simulink model "PaceMaker_Simulink_Model"  (R2018b)
settings: Solver=FixedStepAuto  StartTime=0.0  StopTime=inf  FixedStep=1e-3  RelTol=1e-3  EnableMultiTasking=on
undefined symbols (not defined in the file): A0, A1, D0, D1, D10, D11, D12, D13, D2, D3, D5, D6, D8, D9, PTA0, PTA1, PTA2, PTB2, PTB3, PTB9, PTC16, PTC17, PTC2, PTC4, PTD0, PTD1, PTD2, PTD3
libraries: frdmk64flib x21
(part 1 of 2)
settings Model: ExtModeTrigDuration=5  Creator=elgendya  LastModifiedBy=abdul
settings SolverCC: AutoInsertRateTranBlk=on
settings DataIOCC: LimitDataPoints=on
settings OptimizationCC: PassReuseOutputArgsAs=Individual arguments  MaxStackSize=64
settings DebuggingCC: ParameterTunabilityLossMsg=error  AllowSymbolicDim=off  SFUnexpectedBacktrackingDiag=warning  SFNoUnconditionalDefaultTransitionDiag=warning  SFExecutionAtInitializationDiag=none
settings HardwareCC: ProdBitPerPointer=32  ProdBitPerSizeT=32  ProdBitPerPtrDiffT=32  ProdLargestAtomicInteger=Long  ProdLargestAtomicFloat=Double  ProdWordSize=32  ProdHWDeviceType=ARM Compatible->ARM Cortex
settings SFSimCC: SimUseLocalCustomCode=off  MATLABDynamicMemAlloc=off
settings RTWCC: SystemTargetFile=ert.tlc  HardwareBoard=NXP FRDM-K64F  TLCOptions="-aInlineSetEventsForThisBaseRateFcn=TLC_FALSE -aSuppressMultiTaskScheduler=TLC_FALSE    -aRateBasedStepFcn=0"  TemplateMakefile=ert_default_tmf  GenerateReport=on  RTWUseLocalCustomCode=off  Toolchain=GNU Tools for ARM Embedded Processors  IncludeHyperlinkInReport=on  LaunchReport=on  GenerateTraceInfo=on  GenerateTraceReport=on  GenerateTraceReportSl=on  GenerateTraceReportSf=on  GenerateTraceReportEml=on
settings CodeAppCC: ForceParamTrailComments=on  IgnoreCustomStorageClasses=off  OperatorAnnotations=on  SimulinkDataObjDesc=on  SFDataObjDesc=on  InsertBlockDesc=on
settings ConfigComp: CovMetricSettings=dw  CovHtmlReporting=on  CovSaveCumulativeToWorkspaceVar=on  CovSaveSingleToWorkspaceVar=on  CovShowResultsExplorer=off  CovExternalEMLEnable=off  CovSFcnEnable=off

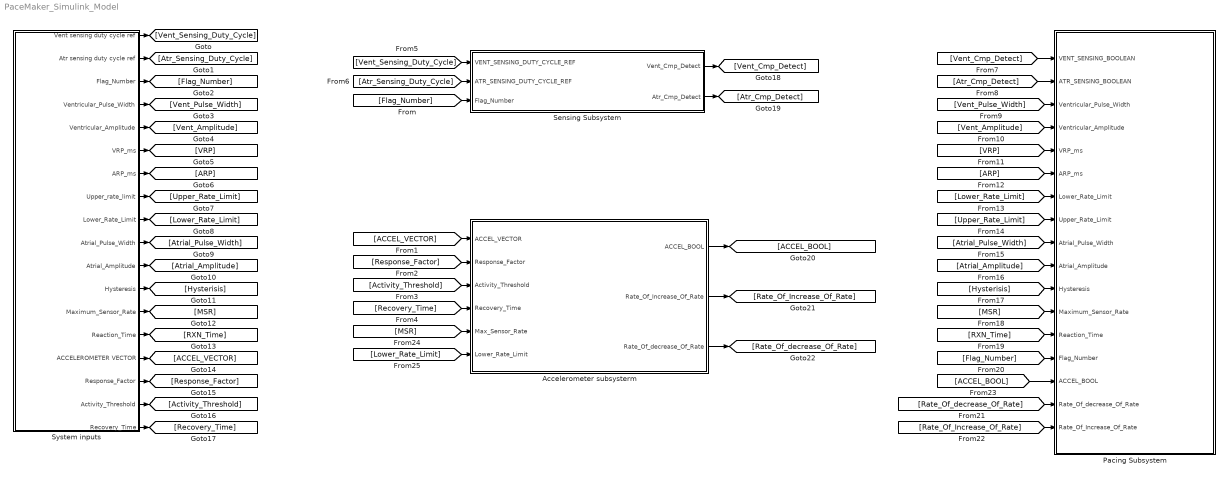
== system PaceMaker_Simulink_Model ==
  "Accelerometer subsysterm " : Subsystem
  "Pacing Subsystem " : Subsystem
  Sensing Subsystem : Subsystem
  "System inputs " : Subsystem
  wires:
  "System inputs "/1(Vent sensing duty cycle ref) -> [Vent_Sensing_Duty_Cycle]
  "System inputs "/2("Atr sensing duty cycle ref ") -> [Atr_Sensing_Duty_Cycle]
  "System inputs "/3(Flag_Number) -> [Flag_Number]
  "System inputs "/4(Ventricular_Pulse_Width) -> [Vent_Pulse_Width]
  "System inputs "/5(Ventricular_Amplitude) -> [Vent_Amplitude]
  "System inputs "/6(VRP_ms) -> [VRP]
  "System inputs "/7(ARP_ms) -> [ARP]
  "System inputs "/8(Upper_rate_limit) -> [Upper_Rate_Limit]
  "System inputs "/9(Lower_Rate_Limit) -> [Lower_Rate_Limit]
  "System inputs "/10(Atrial_Pulse_Width) -> [Atrial_Pulse_Width]
  "System inputs "/11(Atrial_Amplitude) -> [Atrial_Amplitude]
  "System inputs "/12(Hysteresis) -> [Hysterisis]
  "System inputs "/13(Maximum_Sensor_Rate) -> [MSR]
  "System inputs "/14(Reaction_Time) -> [RXN_Time]
  "System inputs "/15(ACCELEROMETER VECTOR) -> [ACCEL_VECTOR]
  "System inputs "/16(Response_Factor) -> [Response_Factor]
  "System inputs "/17(Activity_Threshold) -> [Activity_Threshold]
  "System inputs "/18(Recovery_Time) -> [Recovery_Time]
  [Flag_Number] -> Sensing Subsystem/3(" Flag_Number")
  [ACCEL_VECTOR] -> "Accelerometer subsysterm "/1(ACCEL_VECTOR)
  [Response_Factor] -> "Accelerometer subsysterm "/2(Response_Factor)
  [Activity_Threshold] -> "Accelerometer subsysterm "/3("Activity_Threshold ")
  [Recovery_Time] -> "Accelerometer subsysterm "/4(Recovery_Time)
  [Vent_Sensing_Duty_Cycle] -> Sensing Subsystem/1(" VENT_SENSING_DUTY_CYCLE_REF")
  [Atr_Sensing_Duty_Cycle] -> Sensing Subsystem/2(" ATR_SENSING_DUTY_CYCLE_REF")
  Sensing Subsystem/1(Vent_Cmp_Detect) -> [Vent_Cmp_Detect]
  Sensing Subsystem/2(Atr_Cmp_Detect) -> [Atr_Cmp_Detect]
  [Vent_Cmp_Detect] -> "Pacing Subsystem "/1(VENT_SENSING_BOOLEAN)
  [Atr_Cmp_Detect] -> "Pacing Subsystem "/2(ATR_SENSING_BOOLEAN)
  [Vent_Pulse_Width] -> "Pacing Subsystem "/3(Ventricular_Pulse_Width)
  [Vent_Amplitude] -> "Pacing Subsystem "/4(Ventricular_Amplitude)
  [VRP] -> "Pacing Subsystem "/5(VRP_ms)
  [ARP] -> "Pacing Subsystem "/6(ARP_ms)
  [Lower_Rate_Limit] -> "Pacing Subsystem "/7(Lower_Rate_Limit)
  [Upper_Rate_Limit] -> "Pacing Subsystem "/8(Upper_Rate_Limit)
  [Atrial_Pulse_Width] -> "Pacing Subsystem "/9(Atrial_Pulse_Width)
  [Atrial_Amplitude] -> "Pacing Subsystem "/10(Atrial_Amplitude)
  [Hysterisis] -> "Pacing Subsystem "/11(Hysteresis)
  [MSR] -> "Pacing Subsystem "/12(Maximum_Sensor_Rate)
  [RXN_Time] -> "Pacing Subsystem "/13(Reaction_Time)
  [Flag_Number] -> "Pacing Subsystem "/14(Flag_Number)
  "Accelerometer subsysterm "/1(ACCEL_BOOL) -> [ACCEL_BOOL]
  "Accelerometer subsysterm "/2(Rate_Of_Increase_Of_Rate) -> [Rate_Of_Increase_Of_Rate]
  "Accelerometer subsysterm "/3(Rate_Of_decrease_Of_Rate) -> [Rate_Of_decrease_Of_Rate]
  [Rate_Of_decrease_Of_Rate] -> "Pacing Subsystem "/16(Rate_Of_decrease_Of_Rate)
  [Rate_Of_Increase_Of_Rate] -> "Pacing Subsystem "/17(Rate_Of_Increase_Of_Rate)
  [ACCEL_BOOL] -> "Pacing Subsystem "/15(ACCEL_BOOL)
  [MSR] -> "Accelerometer subsysterm "/5(Max_Sensor_Rate)
  [Lower_Rate_Limit] -> "Accelerometer subsysterm "/6(Lower_Rate_Limit)

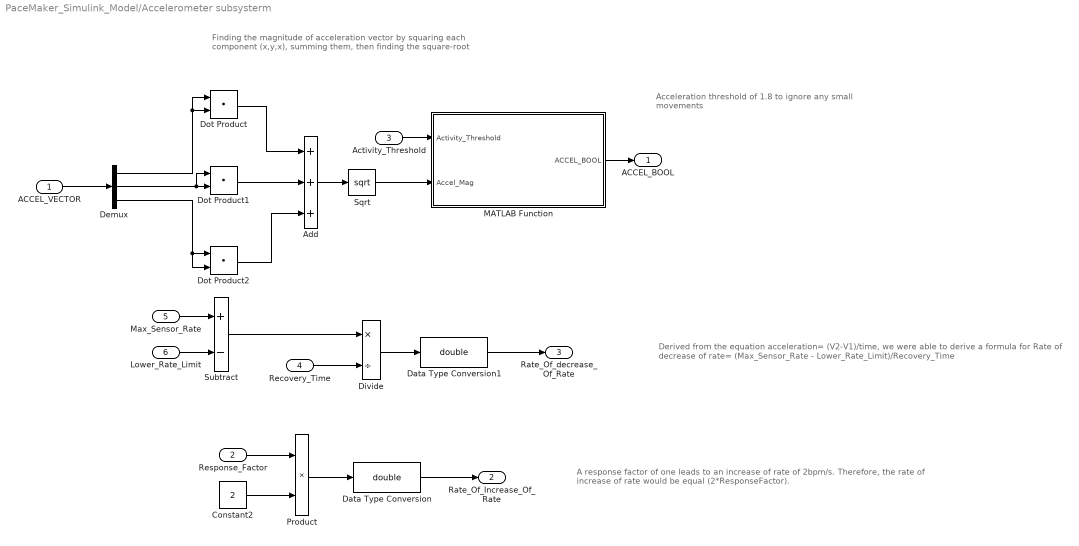
== system PaceMaker_Simulink_Model/Accelerometer subsysterm  ==
  note: Finding the magnitude of acceleration vector by squaring each
      | component (x,y,x), summing them, then finding the square-root
  note: Acceleration threshold of 1.8 to ignore any
      | small movements
  note: A response factor of one leads to an increase of rate of 2bpm/s. Therefore,
      | the rate of increase of rate would be equal (2*ResponseFactor).
  note: Derived from the equation acceleration= (V2-V1)/time, we were able to derive
      | a formula for Rate of decrease of rate= (Max_Sensor_Rate - Lower_Rate_Limit)/Recovery_Time
  ACCEL_VECTOR : Inport
  Response_Factor : Inport  Port=2  OutDataTypeStr=uint16
  "Activity_Threshold " : Inport  Port=3
  Recovery_Time : Inport  Port=4  OutDataTypeStr=uint16
  Max_Sensor_Rate : Inport  Port=5
  Lower_Rate_Limit : Inport  Port=6
  Add : Sum  Inputs=+++
  Constant2 : Constant  Value=2  OutDataTypeStr=uint16
  Data Type Conversion : DataTypeConversion  OutDataTypeStr=double
  Data Type Conversion1 : DataTypeConversion  OutDataTypeStr=double
  Demux : Demux  Outputs=3
  Divide : Product  Inputs=*/
  Dot Product : DotProduct  InputSameDT=on  OutDataTypeStr=Inherit: Inherit via internal rule
  Dot Product1 : DotProduct  InputSameDT=on  OutDataTypeStr=Inherit: Inherit via internal rule
  Dot Product2 : DotProduct  InputSameDT=on  OutDataTypeStr=Inherit: Inherit via internal rule
  MATLAB Function : MATLAB Function  TreatAsAtomicUnit=on
  Product : Product  OutDataTypeStr=uint16
  Sqrt : Sqrt  SaturateOnIntegerOverflow=on
  Subtract : Sum  Inputs=+-
  ACCEL_BOOL : Outport
  Rate_Of_Increase_Of_Rate : Outport  Port=2  OutDataTypeStr=double
  Rate_Of_decrease_Of_Rate : Outport  Port=3  OutDataTypeStr=double
  wires:
  ACCEL_VECTOR/1 -> Demux/1
  Demux/3 -> Dot Product2/1, Dot Product2/2
  Demux/2 -> Dot Product1/1, Dot Product1/2
  Demux/1 -> Dot Product/2, Dot Product/1
  Dot Product1/1 -> Add/2
  Dot Product/1 -> Add/1
  Dot Product2/1 -> Add/3
  Add/1 -> Sqrt/1
  Response_Factor/1 -> Product/1
  Constant2/1 -> Product/2
  "Activity_Threshold "/1 -> MATLAB Function/1(Activity_Threshold)
  Recovery_Time/1 -> Divide/2
  Product/1 -> Data Type Conversion/1
  Data Type Conversion/1 -> Rate_Of_Increase_Of_Rate/1
  Divide/1 -> Data Type Conversion1/1
  Data Type Conversion1/1 -> Rate_Of_decrease_Of_Rate/1
  Lower_Rate_Limit/1 -> Subtract/2
  Max_Sensor_Rate/1 -> Subtract/1
  Subtract/1 -> Divide/1
  Sqrt/1 -> MATLAB Function/2(Accel_Mag)
  MATLAB Function/1(ACCEL_BOOL) -> ACCEL_BOOL/1

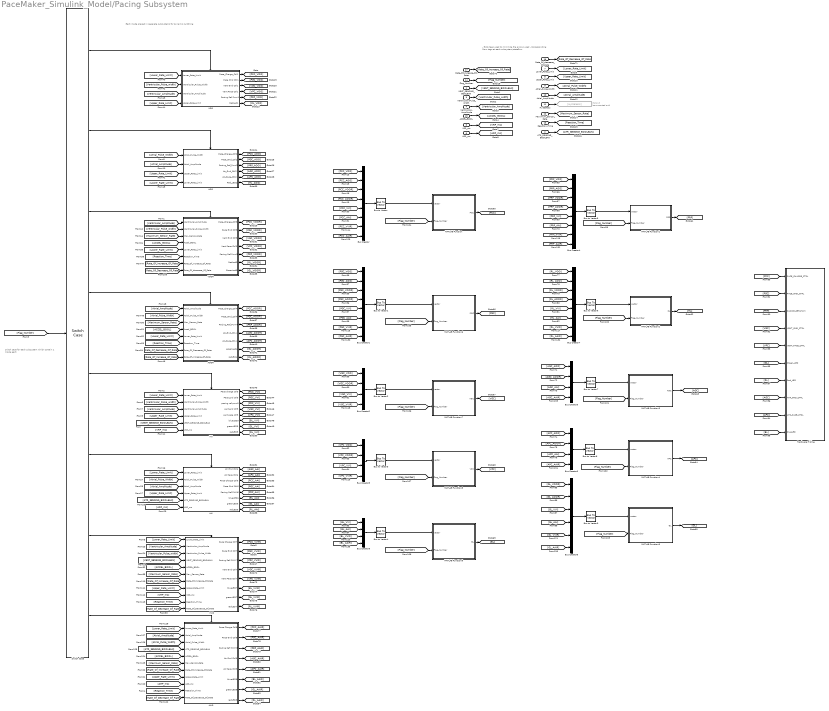
== system PaceMaker_Simulink_Model/Pacing Subsystem  ==
  note: - Goto tags used to minimize the arrows used
      | - Corresponding From tags at each subsystem/stateflow
  note: switch case for each subsystem which contain
      | 1 mode each
  note: Each mode placed in separate subsystems for dynamic switching
  VENT_SENSING_BOOLEAN : Inport
  ATR_SENSING_BOOLEAN : Inport  Port=2
  Ventricular_Pulse_Width : Inport  Port=3
  Ventricular_Amplitude : Inport  Port=4  OutDataTypeStr=uint16
  VRP_ms : Inport  Port=5
  ARP_ms : Inport  Port=6
  Lower_Rate_Limit : Inport  Port=7
  Upper_Rate_Limit : Inport  Port=8
  Atrial_Pulse_Width : Inport  Port=9
  Atrial_Amplitude : Inport  Port=10  OutDataTypeStr=uint16
  Hysteresis : Inport  Port=11
  Maximum_Sensor_Rate : Inport  Port=12
  Reaction_Time : Inport  Port=13
  Flag_Number : Inport  Port=14
  ACCEL_BOOL : Inport  Port=15
  Rate_Of_decrease_Of_Rate : Inport  Port=16
  Rate_Of_Increase_Of_Rate : Inport  Port=17
  AAI : Subsystem  TreatAsAtomicUnit=on
  AAIR : Subsystem  TreatAsAtomicUnit=on
  AOO : Subsystem  TreatAsAtomicUnit=on
  AOOR : Subsystem  TreatAsAtomicUnit=on
  Bus Creator{,1,4,7} (4 alike) : BusCreator  Inputs=8
  Bus Creator{2..3,5..6,9} (5 alike) : BusCreator  Inputs=4
  Bus Creator8 : BusCreator  Inputs=6
  Bus to Vector{,1..9} (10 alike) : BusToVector
  Goto13 : Goto  Commented=on  GotoTag=Hysteresis
  Hardware Hiding : Subsystem  TreatAsAtomicUnit=on
  MATLAB Function : MATLAB Function  TreatAsAtomicUnit=on
  MATLAB Function1 : MATLAB Function  TreatAsAtomicUnit=on
  MATLAB Function2 : MATLAB Function  TreatAsAtomicUnit=on
  MATLAB Function3 : MATLAB Function  TreatAsAtomicUnit=on
  MATLAB Function4 : MATLAB Function  TreatAsAtomicUnit=on
  MATLAB Function5 : MATLAB Function  TreatAsAtomicUnit=on
  MATLAB Function6 : MATLAB Function  TreatAsAtomicUnit=on
  MATLAB Function7 : MATLAB Function  TreatAsAtomicUnit=on
  MATLAB Function8 : MATLAB Function  TreatAsAtomicUnit=on
  MATLAB Function9 : MATLAB Function  TreatAsAtomicUnit=on
  Switch Case : SwitchCase  CaseConditions={1,2,3,4,5,6,7,8,}  ShowDefaultCase=off
  VOO : Subsystem  TreatAsAtomicUnit=on
  VOOR : Subsystem  TreatAsAtomicUnit=on
  "VVI " : Subsystem  TreatAsAtomicUnit=on
  VVIR : Subsystem  TreatAsAtomicUnit=on
  wires:
  VRP_ms/1 -> [VRP_ms]
  ACCEL_BOOL/1 -> [ACCEL_BOOL]
  Ventricular_Amplitude/1 -> [Ventricular_Amplitude]
  Ventricular_Pulse_Width/1 -> [Ventricular_Pulse_width]
  VENT_SENSING_BOOLEAN/1 -> [VENT_SENSING_BOOLEAN]
  ARP_ms/1 -> [ARP_ms]
  Lower_Rate_Limit/1 -> [Lower_Rate_Limit]
  Upper_Rate_Limit/1 -> [Upper_Rate_Limit]
  Atrial_Pulse_Width/1 -> [Atrial_Pulse_Width]
  Atrial_Amplitude/1 -> [Atrial_Amplitude]
  Hysteresis/1 -> Goto13/1
  Maximum_Sensor_Rate/1 -> [Maximum_Sensor_Rate]
  Reaction_Time/1 -> [Reaction_Time]
  Switch Case/1 -> VOO/Action
  Switch Case/2 -> AOO/Action
  Switch Case/4 -> AOOR/Action
  Switch Case/5 -> "VVI "/Action
  Switch Case/6 -> AAI/Action
  Switch Case/7 -> VVIR/Action
  [Lower_Rate_Limit] -> VOO/1(Lower_Rate_LImit)
  [Ventricular_Pulse_width] -> VOO/2(Ventricular_Pulse_Width)
  [Ventricular_Amplitude] -> VOO/3(Ventricular_Amplitude)
  [Upper_Rate_Limit] -> VOO/4(Upper_Rate_Limit)
  [Atrial_Pulse_Width] -> AOO/1(Atrial_Pulse_Width)
  [Atrial_Amplitude] -> AOO/2(Atrial_Amplitude)
  [Lower_Rate_Limit] -> AOO/4(Lower_Rate_Limit)
  [Upper_Rate_Limit] -> AOO/3(Upper_Rate_Limit)
  [Ventricular_Amplitude] -> VOOR/1(Ventricular_Amplitude)
  [Maximum_Sensor_Rate] -> VOOR/3(Max_Sensor_Rate)
  [Ventricular_Pulse_width] -> VOOR/2(Ventricular_Pulse_Width)
  [ACCEL_BOOL] -> VOOR/4(Accel_BOOL)
  [Lower_Rate_Limit] -> VOOR/5(Lower_Rate_Limit)
  [Reaction_Time] -> VOOR/6(Reaction_Time)
  [Atrial_Amplitude] -> AOOR/1(Atrial_Amplitude)
  [Maximum_Sensor_Rate] -> AOOR/3(Max_Sensor_Rate)
  [Atrial_Pulse_Width] -> AOOR/2(Atrial_Pulse_Width)
  [ACCEL_BOOL] -> AOOR/4(Accel_BOOL)
  [Lower_Rate_Limit] -> AOOR/5(Lower_Rate_Limit)
  [Reaction_Time] -> AOOR/6(Reaction_Time)
  [Lower_Rate_Limit] -> "VVI "/1(Lower_Rate_LImit)
  [Ventricular_Pulse_width] -> "VVI "/2(Ventricular_Pulse_Width)
  [Ventricular_Amplitude] -> "VVI "/3(Ventricular_Amplitude)
  [Upper_Rate_Limit] -> "VVI "/4(Upper_Rate_Limit)
  [VENT_SENSING_BOOLEAN] -> "VVI "/5(VENT_SENSING_BOOLEAN)
  [VRP_ms] -> "VVI "/6(VRP_ms)
  ATR_SENSING_BOOLEAN/1 -> [ATR_SENSING_BOOLEAN]
  [Lower_Rate_Limit] -> AAI/1(Lower_Rate_Limit)
  [Upper_Rate_Limit] -> AAI/4(Upper_Rate_Limit)
  [ATR_SENSING_BOOLEAN] -> AAI/5(ATR_SENSING_BOOLEAN)
  [Atrial_Pulse_Width] -> AAI/2(Atrial_Pulse_Width)
  [Atrial_Amplitude] -> AAI/3(Atrial_Amplitude)
  [ARP_ms] -> AAI/6(ARP_ms)
  Flag_Number/1 -> [Flag_Number]
  [Flag_Number] -> Switch Case/1
  VOO/1(Pace_Charge_Ctrl1) -> [PCC_VOO]
  VOO/2(Pace Gnd Ctrl1) -> [PGC_VOO]
  VOO/3(Vent Gnd Ctrl1) -> [VGC_VOO]
  VOO/4(Vent Pace Ctrl1) -> [VPC_VOO]
  VOO/5(Pacing Ref Pwm1) -> [PRP_VOO]
  VOO/6(RedLed1) -> [RL_VOO]
  AOO/1(Pace_Charge_Ctrl2) -> [PCC_AOO]
  AOO/2(Pace_Gnd_Ctrl2) -> [PGC_AOO]
  AOO/3(Pacing_Ref_Pwm2) -> [PRP_AOO]
  AOO/4(Atr_Gnd_Ctrl2) -> [AGC_AOO]
  AOO/5(Atr_Pace_Ctrl2) -> [APC_AOO]
  VOOR/1(Pace_Charge_Ctrl3) -> [PCC_VOOR]
  VOOR/2(Pace Gnd Ctrl3) -> [PGC_VOOR]
  VOOR/3(Vent Gnd Ctrl3) -> [VGC_VOOR]
  VOOR/4(Vent Pace Ctrl3) -> [VPC_VOOR]
  VOOR/5(Pacing Ref Pwm3) -> [PRP_VOOR]
  VOOR/7(GreenLed3) -> [GL_VOOR]
  VOOR/6(RedLed3) -> [RL_VOOR]
  AOOR/1(Pace_Charge_Ctrl4) -> [PCC_AOOR]
  AOOR/2(Pace_Gnd_Ctrl4) -> [PGC_AOOR]
  AOOR/3(Pacing_Ref_Pwm4) -> [PRP_AOOR]
  AOOR/4(Atr_Gnd_Ctrl4) -> [AGC_AOOR]
  AOOR/5(Atr_Pace_Ctrl4) -> [APC_AOOR]
  AOOR/6(greenLed4) -> [GL_AOOR]
  AOOR/7(redLEd4) -> [RL_AOOR]
  "VVI "/1(Pace charge ctrl5) -> [PCC_VVI]
  "VVI "/2(Pace gnd ctrl5) -> [PGC_VVI]
  "VVI "/3(pacing ref pwm5) -> [PRP_VVI]
  "VVI "/4(vent gnd ctrl5) -> [VGC_VVI]
  "VVI "/5(vent pace ctrl5) -> [VPC_VVI]
  "VVI "/6(blueLED5) -> [BL_VVI]
  "VVI "/7(greenLED5) -> [GL_VVI]
  "VVI "/8(redLED5) -> [RL_VVI]
  AAI/1(Atr Gnd Ctrl6) -> [AGC_AAI]
  AAI/2(Atr Pace Ctrl6) -> [APC_AAI]
  AAI/3(Pace Charge Ctrl6) -> [PCC_AAI]
  AAI/5(Pacing Ref PWM6) -> [PRP_AAI]
  AAI/6(blueLED6) -> [BL_AAI]
  AAI/7(greenLED6) -> [GL_AAI]
  AAI/8(redLED6) -> [RL_AAI]
  AAI/4(Pace Gnd Ctrl6) -> [PGC_AAI]
  [PCC_VOO] -> Bus Creator/1
  [PCC_AOO] -> Bus Creator/2
  [PCC_VOOR] -> Bus Creator/3
  [PCC_AOOR] -> Bus Creator/4
  [PCC_VVI] -> Bus Creator/5
  [PCC_AAI] -> Bus Creator/6
  [PGC_AAI] -> Bus Creator1/6
  [PGC_VVI] -> Bus Creator1/5
  [PGC_AOOR] -> Bus Creator1/4
  [PGC_VOOR] -> Bus Creator1/3
  [PGC_AOO] -> Bus Creator1/2
  [PGC_VOO] -> Bus Creator1/1
  [VGC_VOO] -> Bus Creator2/1
  [VGC_VOOR] -> Bus Creator2/2
  [VGC_VVI] -> Bus Creator2/3
  [VPC_VVI] -> Bus Creator3/3
  [VPC_VOOR] -> Bus Creator3/2
  [VPC_VOO] -> Bus Creator3/1
  [PRP_AAI] -> Bus Creator4/6
  [PRP_VVI] -> Bus Creator4/5
  [PRP_AOOR] -> Bus Creator4/4
  [PRP_VOOR] -> Bus Creator4/3
  [PRP_AOO] -> Bus Creator4/2
  [PRP_VOO] -> Bus Creator4/1
  [AGC_AAI] -> Bus Creator5/3
  [AGC_AOOR] -> Bus Creator5/2
  [AGC_AOO] -> Bus Creator5/1
  [APC_AOO] -> Bus Creator6/1
  [APC_AOOR] -> Bus Creator6/2
  [APC_AAI] -> Bus Creator6/3
  AOO/6(Red_LED2) -> [RL_AOO]
  [RL_VOO] -> Bus Creator7/1
  [RL_AOO] -> Bus Creator7/2
  [RL_VOOR] -> Bus Creator7/3
  [RL_AOOR] -> Bus Creator7/4
  [RL_VVI] -> Bus Creator7/5
  [RL_AAI] -> Bus Creator7/6
  [GL_VOOR] -> Bus Creator8/1
  [GL_AOOR] -> Bus Creator8/2
  [GL_VVI] -> Bus Creator8/3
  [GL_AAI] -> Bus Creator8/4
  [BL_VVI] -> Bus Creator9/1
  [BL_AAI] -> Bus Creator9/2
  Bus Creator/1 -> Bus to Vector/1
  Bus Creator1/1 -> Bus to Vector1/1
  Bus Creator2/1 -> Bus to Vector2/1
  Bus Creator3/1 -> Bus to Vector3/1
  Bus Creator9/1 -> Bus to Vector4/1
  Bus Creator4/1 -> Bus to Vector5/1
  Bus Creator7/1 -> Bus to Vector6/1
  Bus Creator5/1 -> Bus to Vector7/1
  Bus Creator6/1 -> Bus to Vector8/1
  Bus Creator8/1 -> Bus to Vector9/1
  Bus to Vector/1 -> MATLAB Function/1(vector)
  MATLAB Function/1(PCC) -> [PCC]
  MATLAB Function1/1(PRP) -> [PRP]
  Bus to Vector5/1 -> MATLAB Function1/1(vector)
  Bus to Vector6/1 -> MATLAB Function2/1(vector)
  MATLAB Function2/1(RL) -> [RL]
  MATLAB Function3/1(AGC) -> [AGC]
  Bus to Vector7/1 -> MATLAB Function3/1(vector)
  Bus to Vector8/1 -> MATLAB Function4/1(vector)
  MATLAB Function4/1(APC) -> [APC]
  MATLAB Function5/1(GL) -> [GL]
  Bus to Vector9/1 -> MATLAB Function5/1(vector)
  [PCC] -> Hardware Hiding/1(PACE_CHARGE_CTRL)
  [PRP] -> Hardware Hiding/3(PACING_REF_PWM)
  [PGC] -> Hardware Hiding/2(PACE_GND_CTRL)
  [VGC] -> Hardware Hiding/4(VENT_GND_CTRL)
  [VPC] -> Hardware Hiding/5(VENT_PACE_CTRL)
  [APC] -> Hardware Hiding/9(ATR_PACE_CTRL)
  [GL] -> Hardware Hiding/6(Green_LED)
  [AGC] -> Hardware Hiding/8(ATR_GND_CTRL)
  [RL] -> Hardware Hiding/7(Red_LED)
  [BL] -> Hardware Hiding/10(blueLED)
  [Flag_Number] -> MATLAB Function1/2(Flag_Number)
  [Flag_Number] -> MATLAB Function2/2(Flag_Number)
  [Flag_Number] -> MATLAB Function3/2(Flag_Number)
  [Flag_Number] -> MATLAB Function4/2(Flag_Number)
  [Flag_Number] -> MATLAB Function5/2(Flag_Number)
  [Flag_Number] -> MATLAB Function/2(Flag_Number)
  [Flag_Number] -> MATLAB Function6/2(Flag_Number)
  MATLAB Function6/1(PGC) -> [PGC]
  Bus to Vector1/1 -> MATLAB Function6/1(vector)
  MATLAB Function7/1(VGC) -> [VGC]
  [Flag_Number] -> MATLAB Function7/2(Flag_Number)
  [Flag_Number] -> MATLAB Function8/2(Flag_Number)
  MATLAB Function8/1(VPC) -> [VPC]
  Bus to Vector3/1 -> MATLAB Function8/1(vector)
  Bus to Vector4/1 -> MATLAB Function9/1(vector)
  MATLAB Function9/1(BL) -> [BL]
  [Flag_Number] -> MATLAB Function9/2(Flag_Number)
  Bus to Vector2/1 -> MATLAB Function7/1(vector)
  [Rate_Of_Increase_Of_Rate] -> VOOR/7(Rate_Of_Increase_Of_Rate)
  [Rate_Of_Decrease_Of_Rate] -> VOOR/8(Rate_Of_decrease_Of_Rate)
  Rate_Of_decrease_Of_Rate/1 -> [Rate_Of_Decrease_Of_Rate]
  Rate_Of_Increase_Of_Rate/1 -> [Rate_Of_Increase_Of_Rate]
  [Rate_Of_Increase_Of_Rate] -> AOOR/8(Rate_Of_increase_Of_Rate)
  [Rate_Of_Decrease_Of_Rate] -> AOOR/7(Rate_Of_Decrease_Of_Rate)
  [Lower_Rate_Limit] -> VVIR/1(Lower_Rate_Limit)
  [Ventricular_Amplitude] -> VVIR/2(Ventricular_Amplitude)
  [Ventricular_Pulse_width] -> VVIR/3(Ventricular_Pulse_Width)
  [VENT_SENSING_BOOLEAN] -> VVIR/4(VENT_SENSING_BOOLEAN)
  [ACCEL_BOOL] -> VVIR/5(ACCEL_BOOL)
  [Maximum_Sensor_Rate] -> VVIR/6(Max_Sensor_Rate)
  [Rate_Of_Increase_Of_Rate] -> VVIR/7(Rate_Of_Increase_Of_Rate)
  [Upper_Rate_Limit] -> VVIR/8(Upper_Rate_Limit)
  [VRP_ms] -> VVIR/9(VRP_ms)
  [Reaction_Time] -> VVIR/10(Reaction_Time)
  VVIR/1(Pace Charge Ctrl7) -> [PCC_VVIR]
  VVIR/2(Pace Gnd Ctrl7) -> [PGC_VVIR]
  VVIR/3(Pacing Ref PWM 7) -> [PRP_VVIR]
  VVIR/4(Vent Gnd Ctrl7) -> [VGC_VVIR]
  VVIR/5(Vent Pace Ctrl7) -> [VPC_VVIR]
  VVIR/6(blueLED7) -> [BL_VVIR]
  VVIR/7(greenLED7) -> [GL_VVIR]
  VVIR/8(redLED7) -> [RL_VVIR]
  [PCC_VVIR] -> Bus Creator/7
  [PGC_VVIR] -> Bus Creator1/7
  [PRP_VVIR] -> Bus Creator4/7
  [RL_VVIR] -> Bus Creator7/7
  [VGC_VVIR] -> Bus Creator2/4
  [VPC_VVIR] -> Bus Creator3/4
  [BL_VVIR] -> Bus Creator9/3
  [GL_VVIR] -> Bus Creator8/5
  Switch Case/3 -> VOOR/Action
  Switch Case/8 -> AAIR/Action
  [Reaction_Time] -> AAIR/10(Reaction_Time)
  [ARP_ms] -> AAIR/9(ARP_ms)
  [Upper_Rate_Limit] -> AAIR/8(Upper_Rate_Limit)
  [Rate_Of_Increase_Of_Rate] -> AAIR/7(Rate_Of_Increase_Of_Rate)
  [Rate_Of_Decrease_Of_Rate] -> VVIR/11(Rate_Of_Decrease_Of_Rate)
  [Rate_Of_Decrease_Of_Rate] -> AAIR/11(Rate_Of_Decrease_Of_Rate)
  [Maximum_Sensor_Rate] -> AAIR/6(Max_Sensor_Rate)
  [ACCEL_BOOL] -> AAIR/5(ACCEL_BOOL)
  [ATR_SENSING_BOOLEAN] -> AAIR/4(ATR_SENSING_BOOLEAN)
  [Atrial_Pulse_Width] -> AAIR/3(Atrial_Pulse_Width)
  [Atrial_Amplitude] -> AAIR/2(Atrial_Amplitude)
  [Lower_Rate_Limit] -> AAIR/1(Lower_Rate_Limit)
  AAIR/1(Pace Charge Ctrl8) -> [PCC_AAIR]
  AAIR/2(Pace Gnd Ctrl8) -> [PGC_AAIR]
  AAIR/3(Pacing Ref PWM 8) -> [PRP_AAIR]
  AAIR/4(Atr Gnd Ctrl8) -> [AGC_AAIR]
  AAIR/5(Atr Pace Ctrl8) -> [APC_AAIR]
  AAIR/6(blueLED8) -> [BL_AAIR]
  AAIR/7(greenLED8) -> [GL_AAIR]
  AAIR/8(redLED8) -> [RL_AAIR]
  [PCC_AAIR] -> Bus Creator/8
  [PGC_AAIR] -> Bus Creator1/8
  [PRP_AAIR] -> Bus Creator4/8
  [RL_AAIR] -> Bus Creator7/8
  [AGC_AAIR] -> Bus Creator5/4
  [APC_AAIR] -> Bus Creator6/4
  [BL_AAIR] -> Bus Creator9/4
  [GL_AAIR] -> Bus Creator8/6

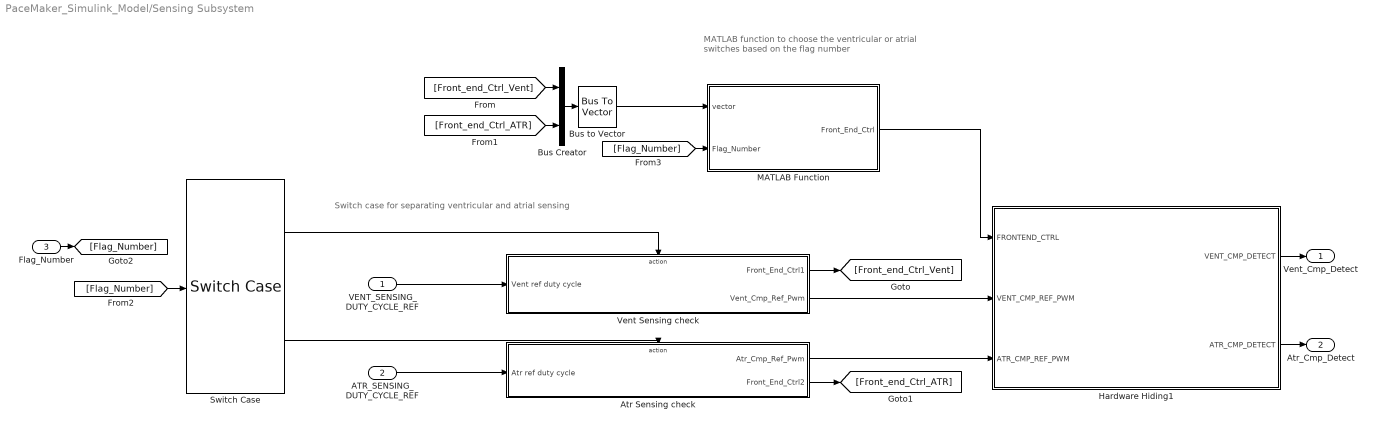
== system PaceMaker_Simulink_Model/Sensing Subsystem ==
  note: Switch case for separating ventricular and atrial sensing
  note: MATLAB function to choose the ventricular or
      | atrial switches based on the flag number
  " VENT_SENSING_DUTY_CYCLE_REF" : Inport
  " ATR_SENSING_DUTY_CYCLE_REF" : Inport  Port=2
  " Flag_Number" : Inport  Port=3
  Atr Sensing check : Subsystem  TreatAsAtomicUnit=on
  Bus Creator : BusCreator  Inputs=2
  Bus to Vector : BusToVector
  Hardware Hiding1 : Subsystem
  MATLAB Function : MATLAB Function  TreatAsAtomicUnit=on
  Switch Case : SwitchCase  CaseConditions={[5,7],[6,8]}  ShowDefaultCase=off
  Vent Sensing check : Subsystem  TreatAsAtomicUnit=on
  Vent_Cmp_Detect : Outport
  Atr_Cmp_Detect : Outport  Port=2
  wires:
  Switch Case/1 -> Vent Sensing check/Action
  " VENT_SENSING_DUTY_CYCLE_REF"/1 -> Vent Sensing check/1("Vent ref duty cycle ")
  Switch Case/2 -> Atr Sensing check/Action
  " ATR_SENSING_DUTY_CYCLE_REF"/1 -> Atr Sensing check/1("Atr ref duty cycle ")
  Vent Sensing check/2(Vent_Cmp_Ref_Pwm) -> Hardware Hiding1/2(VENT_CMP_REF_PWM)
  Hardware Hiding1/1(VENT_CMP_DETECT) -> Vent_Cmp_Detect/1
  Atr Sensing check/1(Atr_Cmp_Ref_Pwm) -> Hardware Hiding1/3(ATR_CMP_REF_PWM)
  Hardware Hiding1/2(ATR_CMP_DETECT) -> Atr_Cmp_Detect/1
  Vent Sensing check/1(Front_End_Ctrl1) -> [Front_end_Ctrl_Vent]
  Atr Sensing check/2(Front_End_Ctrl2) -> [Front_end_Ctrl_ATR]
  [Front_end_Ctrl_Vent] -> Bus Creator/1
  [Front_end_Ctrl_ATR] -> Bus Creator/2
  Bus Creator/1 -> Bus to Vector/1
  Bus to Vector/1 -> MATLAB Function/1(vector)
  " Flag_Number"/1 -> [Flag_Number]
  [Flag_Number] -> Switch Case/1
  [Flag_Number] -> MATLAB Function/2(Flag_Number)
  MATLAB Function/1(Front_End_Ctrl) -> Hardware Hiding1/1("FRONTEND_CTRL ")

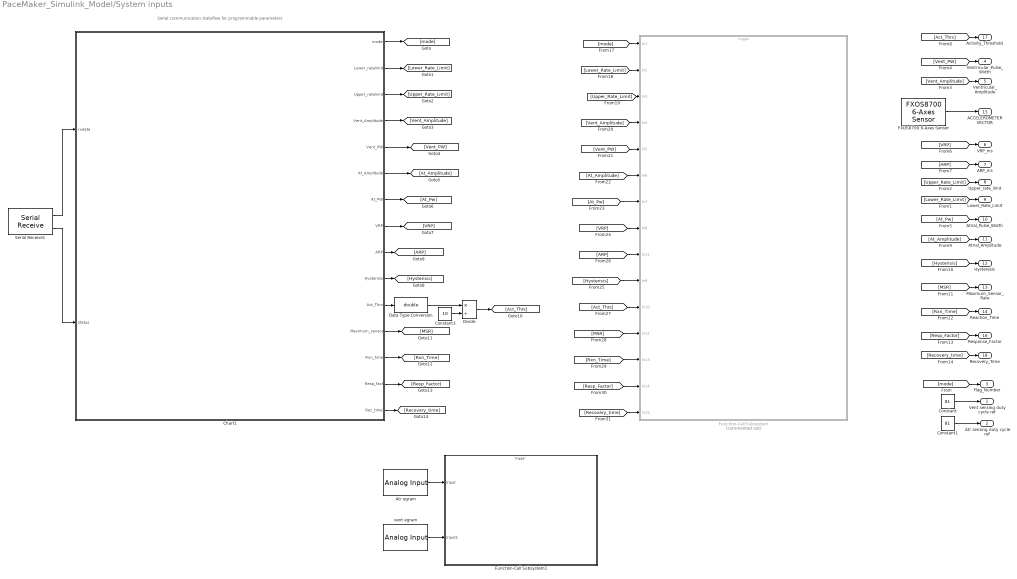
== system PaceMaker_Simulink_Model/System inputs  ==
  note: Serial communication stateflow for programmable parameters
  Atr egram : frdmk64flib/Analog Input  Whichpin=PTB2 (A0)  SampleTime=-1
      settings: SourceProductName=Simulink Coder Support Package for NXP FRDM-K64F Board
  Chart1 : Stateflow chart  TreatAsAtomicUnit=on
  Constant : Constant  Value=81  OutDataTypeStr=uint16
  Constant1 : Constant  Value=81  OutDataTypeStr=uint16
  Constant3 : Constant  Value=10  OutDataTypeStr=double
  Data Type Conversion : DataTypeConversion  OutDataTypeStr=double
  Divide : Product  Inputs=*/
  FXOS8700 6-Axes Sensor : frdmk64flib/FXOS8700 6-Axes Sensor  Activesensor=Accelerometer only  ODR=800Hz  HybridODR=400Hz  Accelfullrange=-4g to +4g  SampleTime=-1
      settings: SourceProductName=Simulink Coder Support Package for NXP FRDM-K64F Board
  Function-Call Subsystem : Subsystem  Commented=on  TreatAsAtomicUnit=on
  Function-Call Subsystem1 : Subsystem  TreatAsAtomicUnit=on
  Serial Receive1 : frdmk64flib/Serial Receive  SCIModule=0  Baudrate=uint32(9600)  Parity=None  StopBits=1  HardwareFlowControl=None  ByteOrder=LittleEndian  DataType=uint16  DataLength=16  BlockingMode=off  OutputStatus=on  SampleTime=-1
      settings: SourceProductName=Simulink Coder Support Package for NXP FRDM-K64F Board
  "vent egram " : frdmk64flib/Analog Input  Whichpin=PTB3 (A1)  SampleTime=-1
      settings: SourceProductName=Simulink Coder Support Package for NXP FRDM-K64F Board
  Vent sensing duty cycle ref : Outport
  "Atr sensing duty cycle ref " : Outport  Port=2
  Flag_Number : Outport  Port=3
  Ventricular_Pulse_Width : Outport  Port=4
  Ventricular_Amplitude : Outport  Port=5
  VRP_ms : Outport  Port=6
  ARP_ms : Outport  Port=7
  Upper_rate_limit : Outport  Port=8  OutDataTypeStr=uint16
  Lower_Rate_Limit : Outport  Port=9
  Atrial_Pulse_Width : Outport  Port=10
  Atrial_Amplitude : Outport  Port=11
  Hysteresis : Outport  Port=12
  Maximum_Sensor_Rate : Outport  Port=13
  Reaction_Time : Outport  Port=14
  ACCELEROMETER VECTOR : Outport  Port=15
  Response_Factor : Outport  Port=16  OutDataTypeStr=uint16
  Activity_Threshold : Outport  Port=17
  Recovery_Time : Outport  Port=18
  wires:
  FXOS8700 6-Axes Sensor/1 -> ACCELEROMETER VECTOR/1
  Serial Receive1/1 -> Chart1/1(rxdata)
  Serial Receive1/2 -> Chart1/2(status)
  Chart1/1(mode) -> [mode]
  Chart1/2(Lower_ratelimit) -> [Lower_Rate_Limit]
  Chart1/3(Upper_ratelimit) -> [Upper_Rate_Limit]
  Chart1/4(Vent_Amplitude) -> [Vent_Amplitude]
  Chart1/5(Vent_PW) -> [Vent_PW]
  Chart1/6(At_Amplitude) -> [At_Amplitude]
  Chart1/7(At_PW) -> [At_Pw]
  Chart1/8(VRP) -> [VRP]
  Chart1/11(Act_Thrs) -> Data Type Conversion/1
  Chart1/12(Maximum_sensor) -> [MSR]
  Chart1/13(Rxn_time) -> [Rxn_Time]
  Chart1/14(Resp_fact) -> [Resp_Factor]
  Chart1/15(Rec_time) -> [Recovery_time]
  [mode] -> Flag_Number/1
  [Lower_Rate_Limit] -> Lower_Rate_Limit/1
  [Upper_Rate_Limit] -> Upper_rate_limit/1
  [Vent_Amplitude] -> Ventricular_Amplitude/1
  [Vent_PW] -> Ventricular_Pulse_Width/1
  [At_Pw] -> Atrial_Pulse_Width/1
  [VRP] -> VRP_ms/1
  [ARP] -> ARP_ms/1
  [Act_Thrs] -> Activity_Threshold/1
  [At_Amplitude] -> Atrial_Amplitude/1
  [Hysterisis] -> Hysteresis/1
  [MSR] -> Maximum_Sensor_Rate/1
  [Rxn_Time] -> Reaction_Time/1
  [Resp_Factor] -> Response_Factor/1
  [Recovery_time] -> Recovery_Time/1
  [mode] -> Function-Call Subsystem/1(In1)
  [Lower_Rate_Limit] -> Function-Call Subsystem/2(In2)
  [Upper_Rate_Limit] -> Function-Call Subsystem/3(In3)
  [Vent_Amplitude] -> Function-Call Subsystem/4(In4)
  [Vent_PW] -> Function-Call Subsystem/5(In5)
  [At_Amplitude] -> Function-Call Subsystem/6(In6)
  [At_Pw] -> Function-Call Subsystem/7(In7)
  [VRP] -> Function-Call Subsystem/8(In8)
  [Act_Thrs] -> Function-Call Subsystem/11(In10)
  [MSR] -> Function-Call Subsystem/12(In12)
  [Rxn_Time] -> Function-Call Subsystem/13(In13)
  [Resp_Factor] -> Function-Call Subsystem/14(In14)
  [Recovery_time] -> Function-Call Subsystem/15(In15)
  Constant/1 -> Vent sensing duty cycle ref/1
  Constant1/1 -> "Atr sensing duty cycle ref "/1
  Chart1/10(Hysterisis) -> [Hysterisis]
  Chart1/9(ARP) -> [ARP]
  [ARP] -> Function-Call Subsystem/9(In11)
  [Hysterisis] -> Function-Call Subsystem/10(In9)
  "vent egram "/1 -> Function-Call Subsystem1/2(Input1)
  Atr egram/1 -> Function-Call Subsystem1/1(Input)
  Divide/1 -> [Act_Thrs]
  Data Type Conversion/1 -> Divide/1
  Constant3/1 -> Divide/2

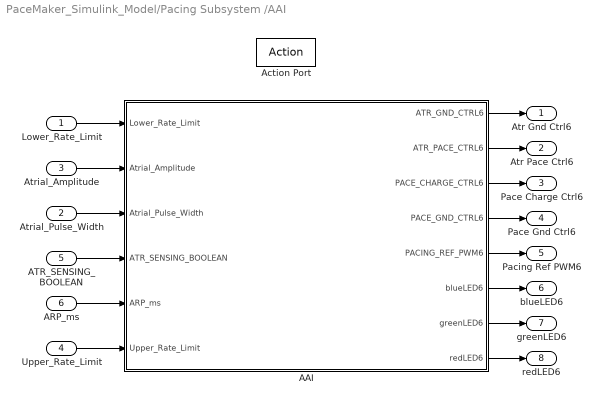
== system PaceMaker_Simulink_Model/Pacing Subsystem /AAI ==
  Lower_Rate_Limit : Inport
  Atrial_Pulse_Width : Inport  Port=2
  Atrial_Amplitude : Inport  Port=3
  Upper_Rate_Limit : Inport  Port=4
  ATR_SENSING_BOOLEAN : Inport  Port=5
  ARP_ms : Inport  Port=6
  Action Port : ActionPort  ActionType=case
  AAI : Stateflow chart  TreatAsAtomicUnit=on
  Atr Gnd Ctrl6 : Outport
  Atr Pace Ctrl6 : Outport  Port=2
  Pace Charge Ctrl6 : Outport  Port=3
  Pace Gnd Ctrl6 : Outport  Port=4
  Pacing Ref PWM6 : Outport  Port=5
  blueLED6 : Outport  Port=6
  greenLED6 : Outport  Port=7
  redLED6 : Outport  Port=8
  wires:
  Lower_Rate_Limit/1 -> AAI/1(Lower_Rate_Limit)
  Atrial_Amplitude/1 -> AAI/2(Atrial_Amplitude)
  Atrial_Pulse_Width/1 -> AAI/3(Atrial_Pulse_Width)
  ATR_SENSING_BOOLEAN/1 -> AAI/4(ATR_SENSING_BOOLEAN)
  ARP_ms/1 -> AAI/5(ARP_ms)
  Upper_Rate_Limit/1 -> AAI/6(Upper_Rate_Limit)
  AAI/1(ATR_GND_CTRL6) -> Atr Gnd Ctrl6/1
  AAI/2(ATR_PACE_CTRL6) -> Atr Pace Ctrl6/1
  AAI/3(PACE_CHARGE_CTRL6) -> Pace Charge Ctrl6/1
  AAI/4(PACE_GND_CTRL6) -> Pace Gnd Ctrl6/1
  AAI/5(PACING_REF_PWM6) -> Pacing Ref PWM6/1
  AAI/6(blueLED6) -> blueLED6/1
  AAI/7(greenLED6) -> greenLED6/1
  AAI/8(redLED6) -> redLED6/1

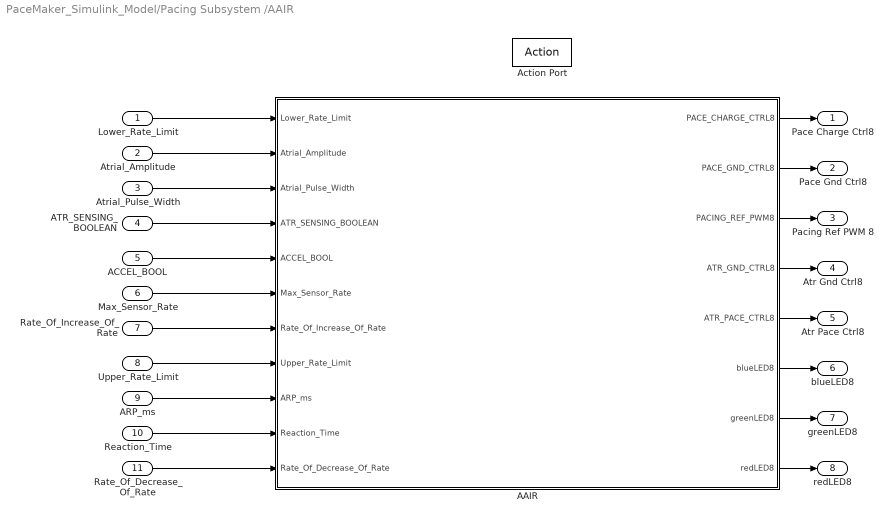
== system PaceMaker_Simulink_Model/Pacing Subsystem /AAIR ==
  Lower_Rate_Limit : Inport
  Atrial_Amplitude : Inport  Port=2
  Atrial_Pulse_Width : Inport  Port=3
  ATR_SENSING_BOOLEAN : Inport  Port=4
  ACCEL_BOOL : Inport  Port=5
  Max_Sensor_Rate : Inport  Port=6
  Rate_Of_Increase_Of_Rate : Inport  Port=7
  Upper_Rate_Limit : Inport  Port=8
  ARP_ms : Inport  Port=9
  Reaction_Time : Inport  Port=10
  Rate_Of_Decrease_Of_Rate : Inport  Port=11
  Action Port : ActionPort  ActionType=case
  AAIR : Stateflow chart  TreatAsAtomicUnit=on
  Pace Charge Ctrl8 : Outport
  Pace Gnd Ctrl8 : Outport  Port=2
  Pacing Ref PWM 8 : Outport  Port=3
  Atr Gnd Ctrl8 : Outport  Port=4
  Atr Pace Ctrl8 : Outport  Port=5
  blueLED8 : Outport  Port=6
  greenLED8 : Outport  Port=7
  redLED8 : Outport  Port=8
  wires:
  ARP_ms/1 -> AAIR/9(ARP_ms)
  Rate_Of_Increase_Of_Rate/1 -> AAIR/7(Rate_Of_Increase_Of_Rate)
  Atrial_Amplitude/1 -> AAIR/2(Atrial_Amplitude)
  Reaction_Time/1 -> AAIR/10(Reaction_Time)
  Upper_Rate_Limit/1 -> AAIR/8(Upper_Rate_Limit)
  ATR_SENSING_BOOLEAN/1 -> AAIR/4(ATR_SENSING_BOOLEAN)
  Max_Sensor_Rate/1 -> AAIR/6(Max_Sensor_Rate)
  ACCEL_BOOL/1 -> AAIR/5(ACCEL_BOOL)
  Atrial_Pulse_Width/1 -> AAIR/3(Atrial_Pulse_Width)
  Lower_Rate_Limit/1 -> AAIR/1(Lower_Rate_Limit)
  AAIR/5(ATR_PACE_CTRL8) -> Atr Pace Ctrl8/1
  AAIR/4(ATR_GND_CTRL8) -> Atr Gnd Ctrl8/1
  AAIR/7(greenLED8) -> greenLED8/1
  AAIR/1(PACE_CHARGE_CTRL8) -> Pace Charge Ctrl8/1
  AAIR/2(PACE_GND_CTRL8) -> Pace Gnd Ctrl8/1
  AAIR/8(redLED8) -> redLED8/1
  AAIR/3(PACING_REF_PWM8) -> Pacing Ref PWM 8/1
  AAIR/6(blueLED8) -> blueLED8/1
  Rate_Of_Decrease_Of_Rate/1 -> AAIR/11(Rate_Of_Decrease_Of_Rate)

== system PaceMaker_Simulink_Model/Pacing Subsystem /AOO ==
  Atrial_Pulse_Width : Inport
  Atrial_Amplitude : Inport  Port=2
  Upper_Rate_Limit : Inport  Port=3
  Lower_Rate_Limit : Inport  Port=4
  Action Port : ActionPort  ActionType=case
  AOO : Stateflow chart  TreatAsAtomicUnit=on
  Pace_Charge_Ctrl2 : Outport
  Pace_Gnd_Ctrl2 : Outport  Port=2
  Pacing_Ref_Pwm2 : Outport  Port=3
  Atr_Gnd_Ctrl2 : Outport  Port=4
  Atr_Pace_Ctrl2 : Outport  Port=5
  Red_LED2 : Outport  Port=6
  wires:
  Atrial_Pulse_Width/1 -> AOO/1(Atrial_Pulse_Width)
  Atrial_Amplitude/1 -> AOO/2(Atrial_Amplitude)
  Lower_Rate_Limit/1 -> AOO/4(Lower_Rate_Limit)
  Upper_Rate_Limit/1 -> AOO/3(Upper_Rate_Limit)
  AOO/1(PACE_CHARGE_CTRL2) -> Pace_Charge_Ctrl2/1
  AOO/2(PACE_GND_CTRL2) -> Pace_Gnd_Ctrl2/1
  AOO/3(PACING_REF_PWM2) -> Pacing_Ref_Pwm2/1
  AOO/4(ATR_GND_CTRL2) -> Atr_Gnd_Ctrl2/1
  AOO/5(ATR_PACE_CTRL2) -> Atr_Pace_Ctrl2/1
  AOO/6(Red_LED2) -> Red_LED2/1

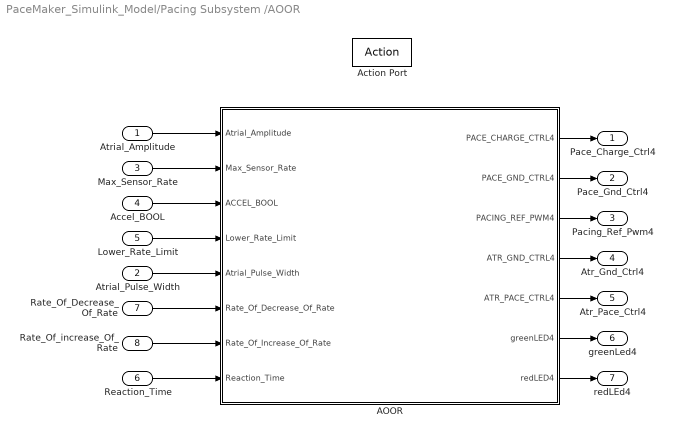
== system PaceMaker_Simulink_Model/Pacing Subsystem /AOOR ==
  Atrial_Amplitude : Inport
  Atrial_Pulse_Width : Inport  Port=2
  Max_Sensor_Rate : Inport  Port=3
  Accel_BOOL : Inport  Port=4
  Lower_Rate_Limit : Inport  Port=5
  Reaction_Time : Inport  Port=6
  Rate_Of_Decrease_Of_Rate : Inport  Port=7
  Rate_Of_increase_Of_Rate : Inport  Port=8
  Action Port : ActionPort  ActionType=case
  AOOR : Stateflow chart  TreatAsAtomicUnit=on
  Pace_Charge_Ctrl4 : Outport
  Pace_Gnd_Ctrl4 : Outport  Port=2
  Pacing_Ref_Pwm4 : Outport  Port=3
  Atr_Gnd_Ctrl4 : Outport  Port=4
  Atr_Pace_Ctrl4 : Outport  Port=5
  greenLed4 : Outport  Port=6
  redLEd4 : Outport  Port=7
  wires:
  AOOR/1(PACE_CHARGE_CTRL4) -> Pace_Charge_Ctrl4/1
  AOOR/2(PACE_GND_CTRL4) -> Pace_Gnd_Ctrl4/1
  AOOR/3(PACING_REF_PWM4) -> Pacing_Ref_Pwm4/1
  AOOR/4(ATR_GND_CTRL4) -> Atr_Gnd_Ctrl4/1
  AOOR/5(ATR_PACE_CTRL4) -> Atr_Pace_Ctrl4/1
  AOOR/6(greenLED4) -> greenLed4/1
  AOOR/7(redLED4) -> redLEd4/1
  Atrial_Amplitude/1 -> AOOR/1(Atrial_Amplitude)
  Reaction_Time/1 -> AOOR/8(Reaction_Time)
  Lower_Rate_Limit/1 -> AOOR/4(Lower_Rate_Limit)
  Max_Sensor_Rate/1 -> AOOR/2(Max_Sensor_Rate)
  Atrial_Pulse_Width/1 -> AOOR/5(Atrial_Pulse_Width)
  Accel_BOOL/1 -> AOOR/3(ACCEL_BOOL)
  Rate_Of_increase_Of_Rate/1 -> AOOR/7(Rate_Of_Increase_Of_Rate)
  Rate_Of_Decrease_Of_Rate/1 -> AOOR/6(Rate_Of_Decrease_Of_Rate)

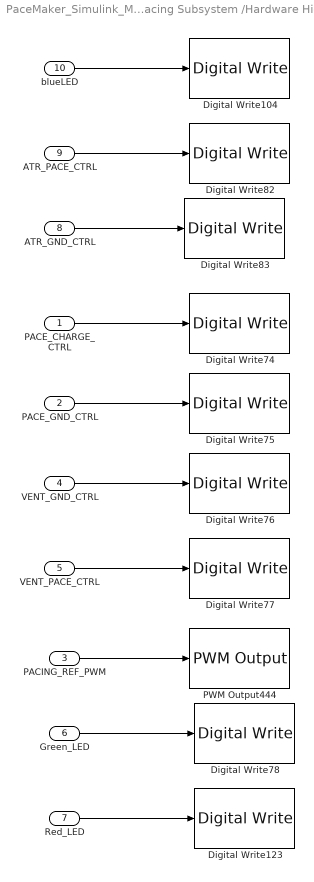
== system PaceMaker_Simulink_Model/Pacing Subsystem /Hardware Hiding ==
  PACE_CHARGE_CTRL : Inport
  PACE_GND_CTRL : Inport  Port=2
  PACING_REF_PWM : Inport  Port=3
  VENT_GND_CTRL : Inport  Port=4
  VENT_PACE_CTRL : Inport  Port=5
  Green_LED : Inport  Port=6
  Red_LED : Inport  Port=7
  ATR_GND_CTRL : Inport  Port=8
  ATR_PACE_CTRL : Inport  Port=9
  blueLED : Inport  Port=10
  Digital Write104 : frdmk64flib/Digital Write  Whichpin=BLUE_LED
      settings: SourceProductName=Simulink Coder Support Package for NXP FRDM-K64F Board
  Digital Write123 : frdmk64flib/Digital Write  Whichpin=RED_LED
      settings: SourceProductName=Simulink Coder Support Package for NXP FRDM-K64F Board
  Digital Write74 : frdmk64flib/Digital Write  Whichpin=PTB9 (D2)
      settings: SourceProductName=Simulink Coder Support Package for NXP FRDM-K64F Board
  Digital Write75 : frdmk64flib/Digital Write  Whichpin=PTD0 (D10)
      settings: SourceProductName=Simulink Coder Support Package for NXP FRDM-K64F Board
  Digital Write76 : frdmk64flib/Digital Write  Whichpin=PTD3 (D12)
      settings: SourceProductName=Simulink Coder Support Package for NXP FRDM-K64F Board
  Digital Write77 : frdmk64flib/Digital Write  Whichpin=PTC4 (D9)
      settings: SourceProductName=Simulink Coder Support Package for NXP FRDM-K64F Board
  Digital Write78 : frdmk64flib/Digital Write  Whichpin=GREEN_LED
      settings: SourceProductName=Simulink Coder Support Package for NXP FRDM-K64F Board
  Digital Write82 : frdmk64flib/Digital Write  Whichpin=PTA0 (D8)
      settings: SourceProductName=Simulink Coder Support Package for NXP FRDM-K64F Board
  Digital Write83 : frdmk64flib/Digital Write  Whichpin=PTD2 (D11)
      settings: SourceProductName=Simulink Coder Support Package for NXP FRDM-K64F Board
  PWM Output444 : frdmk64flib/PWM Output  Whichpin=PTA2 (D5)  InitialFrequency=1000  InitialDutyCycle=0
      settings: SourceProductName=Simulink Coder Support Package for NXP FRDM-K64F Board
  wires:
  Green_LED/1 -> Digital Write78/1
  Red_LED/1 -> Digital Write123/1
  PACING_REF_PWM/1 -> PWM Output444/1
  VENT_GND_CTRL/1 -> Digital Write76/1
  PACE_GND_CTRL/1 -> Digital Write75/1
  PACE_CHARGE_CTRL/1 -> Digital Write74/1
  VENT_PACE_CTRL/1 -> Digital Write77/1
  ATR_PACE_CTRL/1 -> Digital Write82/1
  ATR_GND_CTRL/1 -> Digital Write83/1
  blueLED/1 -> Digital Write104/1

== system PaceMaker_Simulink_Model/Pacing Subsystem /VOO ==
  Lower_Rate_LImit : Inport
  Ventricular_Pulse_Width : Inport  Port=2
  Ventricular_Amplitude : Inport  Port=3
  Upper_Rate_Limit : Inport  Port=4
  Action Port : ActionPort  ActionType=case
  VOO : Stateflow chart  TreatAsAtomicUnit=on
  Pace_Charge_Ctrl1 : Outport
  Pace Gnd Ctrl1 : Outport  Port=2
  Vent Gnd Ctrl1 : Outport  Port=3
  Vent Pace Ctrl1 : Outport  Port=4
  Pacing Ref Pwm1 : Outport  Port=5
  RedLed1 : Outport  Port=6
  wires:
  Lower_Rate_LImit/1 -> VOO/1(Lower_Rate_Limit)
  Ventricular_Pulse_Width/1 -> VOO/2(Ventricular_Pulse_Width)
  Ventricular_Amplitude/1 -> VOO/3(Ventricular_Amplitude)
  Upper_Rate_Limit/1 -> VOO/4(Upper_Rate_Limit)
  VOO/1(PACE_CHARGE_CTRL1) -> Pace_Charge_Ctrl1/1
  VOO/2(PACE_GND_CTRL1) -> Pace Gnd Ctrl1/1
  VOO/3(VENT_GND_CTRL1) -> Vent Gnd Ctrl1/1
  VOO/4(VENT_PACE_CTRL1) -> Vent Pace Ctrl1/1
  VOO/5(PACING_REF_PWM1) -> Pacing Ref Pwm1/1
  VOO/6(RedLED1) -> RedLed1/1

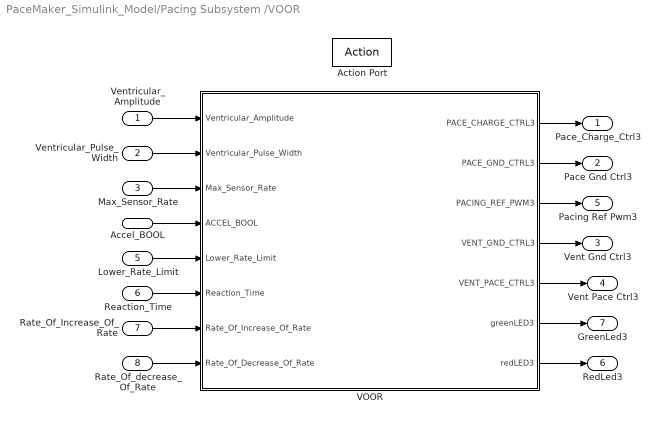
== system PaceMaker_Simulink_Model/Pacing Subsystem /VOOR ==
  Ventricular_Amplitude : Inport
  Ventricular_Pulse_Width : Inport  Port=2
  Max_Sensor_Rate : Inport  Port=3
  Accel_BOOL : Inport  Port=4
  Lower_Rate_Limit : Inport  Port=5
  Reaction_Time : Inport  Port=6
  Rate_Of_Increase_Of_Rate : Inport  Port=7
  Rate_Of_decrease_Of_Rate : Inport  Port=8
  Action Port : ActionPort  ActionType=case
  VOOR : Stateflow chart  TreatAsAtomicUnit=on
  Pace_Charge_Ctrl3 : Outport
  Pace Gnd Ctrl3 : Outport  Port=2
  Vent Gnd Ctrl3 : Outport  Port=3
  Vent Pace Ctrl3 : Outport  Port=4
  Pacing Ref Pwm3 : Outport  Port=5
  RedLed3 : Outport  Port=6
  GreenLed3 : Outport  Port=7
  wires:
  Ventricular_Amplitude/1 -> VOOR/1(Ventricular_Amplitude)
  Ventricular_Pulse_Width/1 -> VOOR/2(Ventricular_Pulse_Width)
  Max_Sensor_Rate/1 -> VOOR/3(Max_Sensor_Rate)
  Accel_BOOL/1 -> VOOR/4(ACCEL_BOOL)
  Lower_Rate_Limit/1 -> VOOR/5(Lower_Rate_Limit)
  Reaction_Time/1 -> VOOR/6(Reaction_Time)
  VOOR/1(PACE_CHARGE_CTRL3) -> Pace_Charge_Ctrl3/1
  VOOR/2(PACE_GND_CTRL3) -> Pace Gnd Ctrl3/1
  VOOR/3(PACING_REF_PWM3) -> Pacing Ref Pwm3/1
  VOOR/4(VENT_GND_CTRL3) -> Vent Gnd Ctrl3/1
  VOOR/5(VENT_PACE_CTRL3) -> Vent Pace Ctrl3/1
  VOOR/6(greenLED3) -> GreenLed3/1
  VOOR/7(redLED3) -> RedLed3/1
  Rate_Of_Increase_Of_Rate/1 -> VOOR/7(Rate_Of_Increase_Of_Rate)
  Rate_Of_decrease_Of_Rate/1 -> VOOR/8(Rate_Of_Decrease_Of_Rate)

== system PaceMaker_Simulink_Model/Pacing Subsystem /VVI  ==
  Lower_Rate_LImit : Inport
  Ventricular_Pulse_Width : Inport  Port=2
  Ventricular_Amplitude : Inport  Port=3
  Upper_Rate_Limit : Inport  Port=4
  VENT_SENSING_BOOLEAN : Inport  Port=5
  VRP_ms : Inport  Port=6
  Action Port : ActionPort  ActionType=case
  VVI : Stateflow chart  TreatAsAtomicUnit=on
  Pace charge ctrl5 : Outport
  Pace gnd ctrl5 : Outport  Port=2
  pacing ref pwm5 : Outport  Port=3
  vent gnd ctrl5 : Outport  Port=4
  vent pace ctrl5 : Outport  Port=5
  blueLED5 : Outport  Port=6
  greenLED5 : Outport  Port=7
  redLED5 : Outport  Port=8
  wires:
  Lower_Rate_LImit/1 -> VVI/1(Lower_Rate_Limit)
  Ventricular_Pulse_Width/1 -> VVI/3(Ventricular_Pulse_Width)
  Ventricular_Amplitude/1 -> VVI/2(Ventricular_Amplitude)
  Upper_Rate_Limit/1 -> VVI/6(Upper_Rate_Limit)
  VRP_ms/1 -> VVI/5(VRP_ms)
  VENT_SENSING_BOOLEAN/1 -> VVI/4(VENT_SENSING_BOOLEAN)
  VVI/1(PACE_CHARGE_CTRL5) -> Pace charge ctrl5/1
  VVI/2(PACE_GND_CTRL5) -> Pace gnd ctrl5/1
  VVI/3(PACING_REF_PWM5) -> pacing ref pwm5/1
  VVI/4(VENT_GND_CTRL5) -> vent gnd ctrl5/1
  VVI/5(VENT_PACE_CTRL5) -> vent pace ctrl5/1
  VVI/6(blueLED5) -> blueLED5/1
  VVI/7(greenLED5) -> greenLED5/1
  VVI/8(redLED5) -> redLED5/1

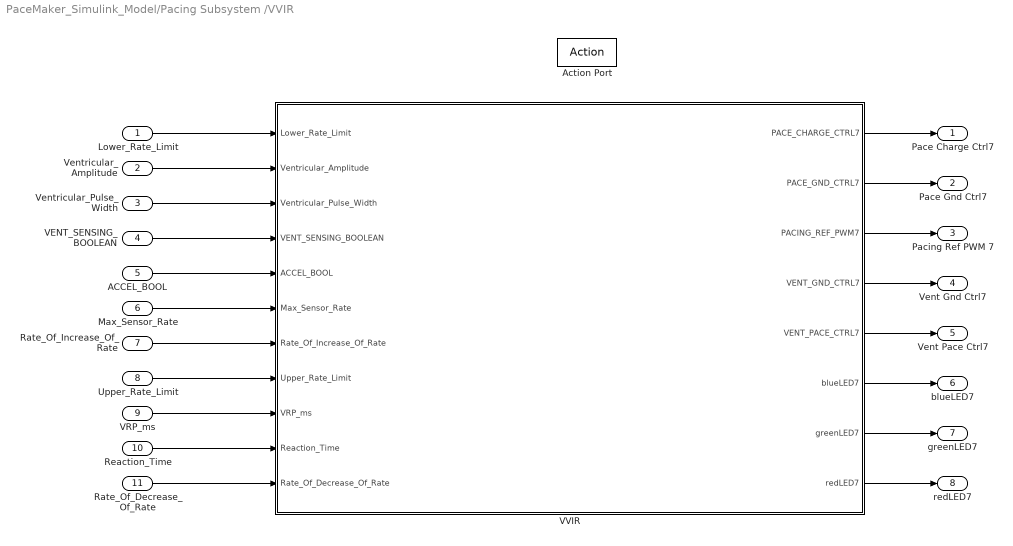
== system PaceMaker_Simulink_Model/Pacing Subsystem /VVIR ==
  Lower_Rate_Limit : Inport
  Ventricular_Amplitude : Inport  Port=2
  Ventricular_Pulse_Width : Inport  Port=3
  VENT_SENSING_BOOLEAN : Inport  Port=4
  ACCEL_BOOL : Inport  Port=5
  Max_Sensor_Rate : Inport  Port=6
  Rate_Of_Increase_Of_Rate : Inport  Port=7
  Upper_Rate_Limit : Inport  Port=8
  VRP_ms : Inport  Port=9
  Reaction_Time : Inport  Port=10
  Rate_Of_Decrease_Of_Rate : Inport  Port=11
  Action Port : ActionPort  ActionType=case
  VVIR : Stateflow chart  TreatAsAtomicUnit=on
  Pace Charge Ctrl7 : Outport
  Pace Gnd Ctrl7 : Outport  Port=2
  Pacing Ref PWM 7 : Outport  Port=3
  Vent Gnd Ctrl7 : Outport  Port=4
  Vent Pace Ctrl7 : Outport  Port=5
  blueLED7 : Outport  Port=6
  greenLED7 : Outport  Port=7
  redLED7 : Outport  Port=8
  wires:
  Lower_Rate_Limit/1 -> VVIR/1(Lower_Rate_Limit)
  Ventricular_Amplitude/1 -> VVIR/2(Ventricular_Amplitude)
  Ventricular_Pulse_Width/1 -> VVIR/3(Ventricular_Pulse_Width)
  VENT_SENSING_BOOLEAN/1 -> VVIR/4(VENT_SENSING_BOOLEAN)
  ACCEL_BOOL/1 -> VVIR/5(ACCEL_BOOL)
  Max_Sensor_Rate/1 -> VVIR/6(Max_Sensor_Rate)
  Rate_Of_Increase_Of_Rate/1 -> VVIR/7(Rate_Of_Increase_Of_Rate)
  Upper_Rate_Limit/1 -> VVIR/8(Upper_Rate_Limit)
  VRP_ms/1 -> VVIR/9(VRP_ms)
  Reaction_Time/1 -> VVIR/10(Reaction_Time)
  VVIR/1(PACE_CHARGE_CTRL7) -> Pace Charge Ctrl7/1
  VVIR/8(redLED7) -> redLED7/1
  VVIR/7(greenLED7) -> greenLED7/1
  VVIR/6(blueLED7) -> blueLED7/1
  VVIR/5(VENT_PACE_CTRL7) -> Vent Pace Ctrl7/1
  VVIR/3(PACING_REF_PWM7) -> Pacing Ref PWM 7/1
  VVIR/2(PACE_GND_CTRL7) -> Pace Gnd Ctrl7/1
  VVIR/4(VENT_GND_CTRL7) -> Vent Gnd Ctrl7/1
  Rate_Of_Decrease_Of_Rate/1 -> VVIR/11(Rate_Of_Decrease_Of_Rate)

== system PaceMaker_Simulink_Model/Sensing Subsystem/Atr Sensing check ==
  "Atr ref duty cycle " : Inport
  Action Port : ActionPort  ActionType=case
  Atr Sensing check : Stateflow chart  TreatAsAtomicUnit=on
  Atr_Cmp_Ref_Pwm : Outport
  Front_End_Ctrl2 : Outport  Port=2
  wires:
  "Atr ref duty cycle "/1 -> Atr Sensing check/1(REF_PWM_DUTY_CYCLE)
  Atr Sensing check/2(Atr_CMP_REF_PWM) -> Atr_Cmp_Ref_Pwm/1
  Atr Sensing check/1(FRONTEND_CTRL2) -> Front_End_Ctrl2/1

== system PaceMaker_Simulink_Model/Sensing Subsystem/Hardware Hiding1 ==
  "FRONTEND_CTRL " : Inport
  VENT_CMP_REF_PWM : Inport  Port=2
  ATR_CMP_REF_PWM : Inport  Port=3
  Digital Read : frdmk64flib/Digital Read  Whichpin=PTC17 (D1)  SampleTime=-1
      settings: SourceProductName=Simulink Coder Support Package for NXP FRDM-K64F Board
  Digital Read1 : frdmk64flib/Digital Read  Whichpin=PTC16 (D0)  SampleTime=-1
      settings: SourceProductName=Simulink Coder Support Package for NXP FRDM-K64F Board
  Digital Write : frdmk64flib/Digital Write  Whichpin=PTD1 (D13)
      settings: SourceProductName=Simulink Coder Support Package for NXP FRDM-K64F Board
  PWM Output : frdmk64flib/PWM Output  Whichpin=PTA1 (D3)  InitialFrequency=1000  InitialDutyCycle=0
      settings: SourceProductName=Simulink Coder Support Package for NXP FRDM-K64F Board
  PWM Output1 : frdmk64flib/PWM Output  Whichpin=PTC2 (D6)  InitialFrequency=1000  InitialDutyCycle=0
      settings: SourceProductName=Simulink Coder Support Package for NXP FRDM-K64F Board
  VENT_CMP_DETECT : Outport
  ATR_CMP_DETECT : Outport  Port=2
  wires:
  VENT_CMP_REF_PWM/1 -> PWM Output/1
  "FRONTEND_CTRL "/1 -> Digital Write/1
  Digital Read/1 -> VENT_CMP_DETECT/1
  Digital Read1/1 -> ATR_CMP_DETECT/1
  ATR_CMP_REF_PWM/1 -> PWM Output1/1

== system PaceMaker_Simulink_Model/Sensing Subsystem/Vent Sensing check ==
  "Vent ref duty cycle " : Inport
  Action Port : ActionPort  ActionType=case
  vent Sensing check : Stateflow chart  TreatAsAtomicUnit=on
  Front_End_Ctrl1 : Outport
  Vent_Cmp_Ref_Pwm : Outport  Port=2
  wires:
  "Vent ref duty cycle "/1 -> vent Sensing check/1(REF_PWM_DUTY_CYCLE)
  vent Sensing check/1(FRONTEND_CTRL1) -> Front_End_Ctrl1/1
  vent Sensing check/2(VENT_CMP_REF_PWM) -> Vent_Cmp_Ref_Pwm/1

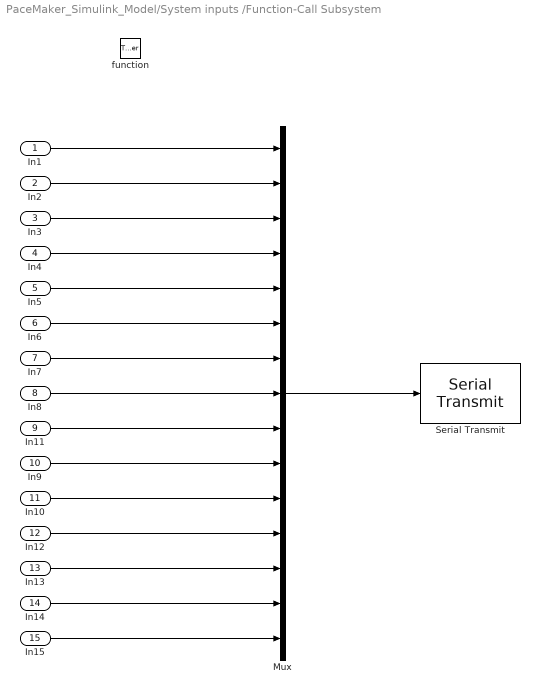
== system PaceMaker_Simulink_Model/System inputs /Function-Call Subsystem ==
  In1 : Inport
  In2 : Inport  Port=2
  In3 : Inport  Port=3
  In4 : Inport  Port=4
  In5 : Inport  Port=5
  In6 : Inport  Port=6
  In7 : Inport  Port=7
  In8 : Inport  Port=8
  In11 : Inport  Port=9
  In9 : Inport  Port=10
  In10 : Inport  Port=11
  In12 : Inport  Port=12
  In13 : Inport  Port=13
  In14 : Inport  Port=14
  In15 : Inport  Port=15
  function : TriggerPort  TriggerType=function-call  IsSimulinkFunction=on  FunctionName=send_param  VariantControl=Variant
  Mux : Mux  Inputs=15
  Serial Transmit : frdmk64flib/Serial Transmit  SCIModule=0  Baudrate=uint32(9600)  Parity=None  StopBits=1  HardwareFlowControl=None  ByteOrder=LittleEndian  BlockingMode=on  OutputStatus=off
      settings: SourceProductName=Simulink Coder Support Package for NXP FRDM-K64F Board
  wires:
  In1/1 -> Mux/1
  In2/1 -> Mux/2
  In3/1 -> Mux/3
  In4/1 -> Mux/4
  In5/1 -> Mux/5
  In6/1 -> Mux/6
  In7/1 -> Mux/7
  In8/1 -> Mux/8
  In11/1 -> Mux/9
  In9/1 -> Mux/10
  In10/1 -> Mux/11
  In12/1 -> Mux/12
  In13/1 -> Mux/13
  In14/1 -> Mux/14
  Mux/1 -> Serial Transmit/1
  In15/1 -> Mux/15

== system PaceMaker_Simulink_Model/System inputs /Function-Call Subsystem1 ==
  Input : Inport
  Input1 : Inport  Port=2
  send_egram : TriggerPort  TriggerType=function-call  IsSimulinkFunction=on  FunctionName=send_egram  VariantControl=Variant
  Data Type Conversion : DataTypeConversion  OutDataTypeStr=double
  Data Type Conversion1 : DataTypeConversion  OutDataTypeStr=double
  Mux : Mux  Inputs=2
  Serial Transmit : frdmk64flib/Serial Transmit  SCIModule=0  Baudrate=uint32(9600)  Parity=None  StopBits=1  HardwareFlowControl=None  ByteOrder=LittleEndian  BlockingMode=on  OutputStatus=off
      settings: SourceProductName=Simulink Coder Support Package for NXP FRDM-K64F Board
  wires:
  Mux/1 -> Serial Transmit/1
  Input/1 -> Data Type Conversion/1
  Input1/1 -> Data Type Conversion1/1
  Data Type Conversion/1 -> Mux/1
  Data Type Conversion1/1 -> Mux/2

== stateflow chart PaceMaker_Simulink_Model/Sensing Subsystem/Atr Sensing check/Atr Sensing check ==
  state Sensing_
    entry:
    FRONTEND_CTRL2=true;
    Atr_CMP_REF_PWM=REF_PWM_DUTY_CYCLE;
  (default) -> Sensing_
  data: FRONTEND_CTRL2 output boolean; Atr_CMP_REF_PWM output uint16; REF_PWM_DUTY_CYCLE input uint16

== stateflow chart PaceMaker_Simulink_Model/Pacing Subsystem /VOOR/VOOR ==
  note: - Using local variable "rate" to control
      | increasing/decreasing pulsing rate
      | - Initializing "rate" to the Lower_Rate_Limit
  state INITIAL
    entry:
    rate=double(Lower_Rate_Limit);
    time=0;
  state Discharging_C22_and_charging_C21
    entry:
    PACE_CHARGE_CTRL3=false;
    VENT_GND_CTRL3=false;
    PACE_GND_CTRL3=true;
    VENT_PACE_CTRL3=true;
    redLED3=true;
    greenLED3=false;
  state Charging_C22_and_Discharging_C21
    entry:
    VENT_PACE_CTRL3=false;
    PACE_CHARGE_CTRL3=true;
    VENT_GND_CTRL3=true;
    PACE_GND_CTRL3=true;
    PACING_REF_PWM3=Ventricular_Amplitude;
    redLED3=false;
    greenLED3=false;
    %time=time+(60/rate);
  state Pace_slower
    entry:
    rate=rate-(Rate_Of_Decrease_Of_Rate)*(60/rate);
    redLED3=false;
    greenLED3=true;
    if rate<Lower_Rate_Limit
    rate=double(60);
    else
    rate=rate;
    end
  state Pace_faster
    entry:
    rate=rate+(Rate_Of_Increase_Of_Rate)*double(60/rate);
    redLED3=false;
    greenLED3=false;
    if rate>Max_Sensor_Rate
    rate=double(120);
    else
    rate=rate;
    end
  Charging_C22_and_Discharging_C21 -> Discharging_C22_and_charging_C21 [order 1] : [after(((60000/rate)-Ventricular_Pulse_Width-10),msec)]{time=time+(60/rate)}
  (default) -> INITIAL
  INITIAL -> Charging_C22_and_Discharging_C21
  Discharging_C22_and_charging_C21 -> (junction 96) : [after(Ventricular_Pulse_Width,msec)]
  (junction 96) -> Charging_C22_and_Discharging_C21 [order 1] : [ACCEL_BOOL == true]
  (junction 96) -> (junction 95) [order 2] : [ACCEL_BOOL == false]{time=0}
  Pace_slower -> Charging_C22_and_Discharging_C21 : [after(10,msec)]
  (junction 95) -> Pace_slower [order 2] : [rate > Lower_Rate_Limit]
  (junction 95) -> Charging_C22_and_Discharging_C21 [order 1] : [rate <= Lower_Rate_Limit]
  (junction 89) -> Discharging_C22_and_charging_C21 : [after(((60000/rate)-Ventricular_Pulse_Width),msec)]
  Pace_faster -> Discharging_C22_and_charging_C21 : [after(((60000/rate)-Ventricular_Pulse_Width),msec)]
  Charging_C22_and_Discharging_C21 -> (junction 99) [order 2] : [(time>Reaction_Time) && (ACCEL_BOOL == true)]
  (junction 99) -> Pace_faster [order 2] : [(rate < Max_Sensor_Rate)]
  (junction 99) -> (junction 89) [order 1] : [rate >= Max_Sensor_Rate]
  data: PACE_CHARGE_CTRL3 output boolean; PACE_GND_CTRL3 output boolean; PACING_REF_PWM3 output uint16; VENT_GND_CTRL3 output boolean; VENT_PACE_CTRL3 output boolean; Ventricular_Amplitude input uint16; Ventricular_Pulse_Width input uint16; Max_Sensor_Rate input uint16; ACCEL_BOOL input boolean; rate local double; greenLED3 output boolean; redLED3 output boolean; Lower_Rate_Limit input uint16; Reaction_Time input uint16; Rate_Of_Increase_Of_Rate input double; time local double; Rate_Of_Decrease_Of_Rate input double

== stateflow chart PaceMaker_Simulink_Model/Pacing Subsystem /VOO/VOO ==
  state Discharging_C22_and_charging_C21
    entry:
    PACE_CHARGE_CTRL1=false;
    VENT_GND_CTRL1=false;
    PACE_GND_CTRL1=true;
    VENT_PACE_CTRL1=true;
    RedLED1=false;
  state Charging_C22_and_Discharging_C21
    entry:
    VENT_PACE_CTRL1=false;
    PACE_CHARGE_CTRL1=true;
    VENT_GND_CTRL1=true;
    PACE_GND_CTRL1=true;
    RedLED1=true;
    PACING_REF_PWM1=Ventricular_Amplitude;
    Upper_Rate_Limit;
  note: Red LED used for on-board testing
  (default) -> Charging_C22_and_Discharging_C21
  Discharging_C22_and_charging_C21 -> Charging_C22_and_Discharging_C21 : [after(Ventricular_Pulse_Width,msec)]
  Charging_C22_and_Discharging_C21 -> Discharging_C22_and_charging_C21 : [after(((60000/Lower_Rate_Limit)-Ventricular_Pulse_Width),msec)]
  data: Lower_Rate_Limit input uint16; PACE_CHARGE_CTRL1 output; PACE_GND_CTRL1 output; VENT_GND_CTRL1 output boolean; VENT_PACE_CTRL1 output boolean; Ventricular_Pulse_Width input uint16; Ventricular_Amplitude input uint16; PACING_REF_PWM1 output uint16; RedLED1 output boolean; Upper_Rate_Limit input uint16

== stateflow chart PaceMaker_Simulink_Model/Sensing Subsystem/Vent Sensing check/vent Sensing check ==
  state Sensing_
    entry:
    FRONTEND_CTRL1=true;
    VENT_CMP_REF_PWM=REF_PWM_DUTY_CYCLE;
  (default) -> Sensing_
  data: FRONTEND_CTRL1 output boolean; VENT_CMP_REF_PWM output uint16; REF_PWM_DUTY_CYCLE input uint16

== stateflow chart PaceMaker_Simulink_Model/Pacing Subsystem /AOO/AOO ==
  note: Red LED used for on-board testing
  state Discharging_C22_and_charging_C21
    entry:
    PACE_CHARGE_CTRL2=false;
    ATR_GND_CTRL2=false;
    PACE_GND_CTRL2=true;
    ATR_PACE_CTRL2=true;
    Red_LED2=false;
  state Charging_C22_and_Discharging_C21
    entry:
    ATR_PACE_CTRL2=false;
    PACE_CHARGE_CTRL2=true;
    ATR_GND_CTRL2=true;
    PACE_GND_CTRL2=true;
    PACING_REF_PWM2=Atrial_Amplitude;
    Red_LED2=true;
    Upper_Rate_Limit;
  (default) -> Charging_C22_and_Discharging_C21
  Discharging_C22_and_charging_C21 -> Charging_C22_and_Discharging_C21 : [after(Atrial_Pulse_Width,msec)]
  Charging_C22_and_Discharging_C21 -> Discharging_C22_and_charging_C21 : [after(((60000/Lower_Rate_Limit)-Atrial_Pulse_Width),msec)]
  data: PACE_CHARGE_CTRL2 output; PACE_GND_CTRL2 output; Atrial_Pulse_Width input uint16; Atrial_Amplitude input uint16; PACING_REF_PWM2 output uint16; ATR_GND_CTRL2 output boolean; ATR_PACE_CTRL2 output boolean; Upper_Rate_Limit input uint16; Lower_Rate_Limit input uint16; Red_LED2 output boolean
